simulink model "Motor_Fault_System"  (R2025b)
settings: Solver=ode4  StartTime=0.0  StopTime=30  FixedStep=0.01  RelTol=1e-3
settings Model: Creator=anifa  LastModifiedBy=anifa

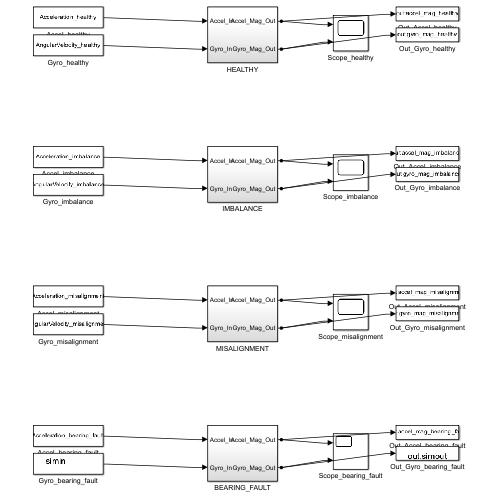
[thumbnail: Simulink's stored preview of the top-level diagram]
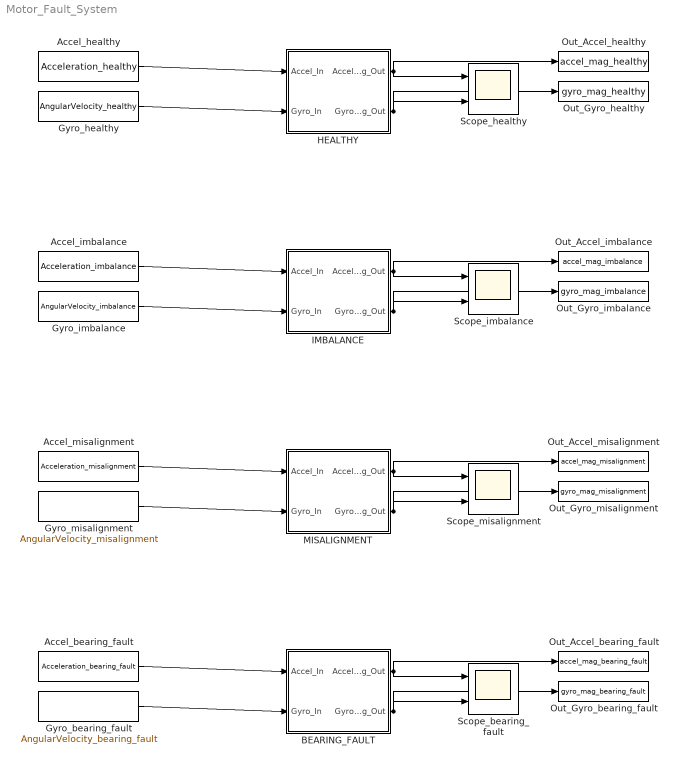
== system Motor_Fault_System ==
  Accel_bearing_fault : FromWorkspace  VariableName=Acceleration_bearing_fault
  Accel_healthy : FromWorkspace  VariableName=Acceleration_healthy
  Accel_imbalance : FromWorkspace  VariableName=Acceleration_imbalance
  Accel_misalignment : FromWorkspace  VariableName=Acceleration_misalignment
  BEARING_FAULT : Subsystem
  Gyro_bearing_fault : FromWorkspace  VariableName=AngularVelocity_bearing_fault
  Gyro_healthy : FromWorkspace  VariableName=AngularVelocity_healthy
  Gyro_imbalance : FromWorkspace  VariableName=AngularVelocity_imbalance
  Gyro_misalignment : FromWorkspace  VariableName=AngularVelocity_misalignment
  HEALTHY : Subsystem
  IMBALANCE : Subsystem
  MISALIGNMENT : Subsystem
  Out_Accel_bearing_fault : ToWorkspace  VariableName=accel_mag_bearing_fault  SampleTime=-1
  Out_Accel_healthy : ToWorkspace  VariableName=accel_mag_healthy  SampleTime=-1
  Out_Accel_imbalance : ToWorkspace  VariableName=accel_mag_imbalance  SampleTime=-1
  Out_Accel_misalignment : ToWorkspace  VariableName=accel_mag_misalignment  SampleTime=-1
  Out_Gyro_bearing_fault : ToWorkspace  VariableName=gyro_mag_bearing_fault  SampleTime=-1
  Out_Gyro_healthy : ToWorkspace  VariableName=gyro_mag_healthy  SampleTime=-1
  Out_Gyro_imbalance : ToWorkspace  VariableName=gyro_mag_imbalance  SampleTime=-1
  Out_Gyro_misalignment : ToWorkspace  VariableName=gyro_mag_misalignment  SampleTime=-1
  Scope_bearing_fault : Scope  NumInputPorts=2
  Scope_healthy : Scope  NumInputPorts=2
  Scope_imbalance : Scope  NumInputPorts=2
  Scope_misalignment : Scope  NumInputPorts=2
  wires:
  Accel_healthy/1 -> HEALTHY/1(Accel_In)
  Gyro_healthy/1 -> HEALTHY/2(Gyro_In)
  HEALTHY/1(Accel_Mag_Out) -> Scope_healthy/1, Out_Accel_healthy/1
  HEALTHY/2(Gyro_Mag_Out) -> Scope_healthy/2, Out_Gyro_healthy/1
  Accel_imbalance/1 -> IMBALANCE/1(Accel_In)
  Gyro_imbalance/1 -> IMBALANCE/2(Gyro_In)
  IMBALANCE/1(Accel_Mag_Out) -> Scope_imbalance/1, Out_Accel_imbalance/1
  IMBALANCE/2(Gyro_Mag_Out) -> Scope_imbalance/2, Out_Gyro_imbalance/1
  Accel_misalignment/1 -> MISALIGNMENT/1(Accel_In)
  Gyro_misalignment/1 -> MISALIGNMENT/2(Gyro_In)
  MISALIGNMENT/1(Accel_Mag_Out) -> Scope_misalignment/1, Out_Accel_misalignment/1
  MISALIGNMENT/2(Gyro_Mag_Out) -> Scope_misalignment/2, Out_Gyro_misalignment/1
  Accel_bearing_fault/1 -> BEARING_FAULT/1(Accel_In)
  Gyro_bearing_fault/1 -> BEARING_FAULT/2(Gyro_In)
  BEARING_FAULT/1(Accel_Mag_Out) -> Scope_bearing_fault/1, Out_Accel_bearing_fault/1
  BEARING_FAULT/2(Gyro_Mag_Out) -> Scope_bearing_fault/2, Out_Gyro_bearing_fault/1

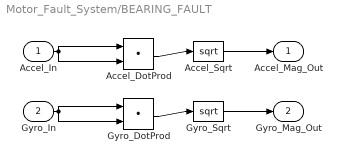
== system Motor_Fault_System/BEARING_FAULT ==
  Accel_In : Inport
  Gyro_In : Inport  Port=2
  Accel_DotProd : DotProduct  OutDataTypeStr=Inherit: Inherit via internal rule
  Accel_Sqrt : Sqrt
  Gyro_DotProd : DotProduct  OutDataTypeStr=Inherit: Inherit via internal rule
  Gyro_Sqrt : Sqrt
  Accel_Mag_Out : Outport
  Gyro_Mag_Out : Outport  Port=2
  wires:
  Accel_In/1 -> Accel_DotProd/1, Accel_DotProd/2
  Accel_DotProd/1 -> Accel_Sqrt/1
  Accel_Sqrt/1 -> Accel_Mag_Out/1
  Gyro_In/1 -> Gyro_DotProd/1, Gyro_DotProd/2
  Gyro_DotProd/1 -> Gyro_Sqrt/1
  Gyro_Sqrt/1 -> Gyro_Mag_Out/1

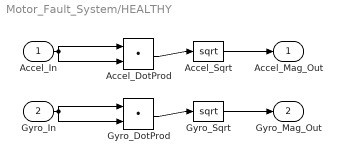
== system Motor_Fault_System/HEALTHY ==
  Accel_In : Inport
  Gyro_In : Inport  Port=2
  Accel_DotProd : DotProduct  OutDataTypeStr=Inherit: Inherit via internal rule
  Accel_Sqrt : Sqrt
  Gyro_DotProd : DotProduct  OutDataTypeStr=Inherit: Inherit via internal rule
  Gyro_Sqrt : Sqrt
  Accel_Mag_Out : Outport
  Gyro_Mag_Out : Outport  Port=2
  wires:
  Accel_In/1 -> Accel_DotProd/1, Accel_DotProd/2
  Accel_DotProd/1 -> Accel_Sqrt/1
  Accel_Sqrt/1 -> Accel_Mag_Out/1
  Gyro_In/1 -> Gyro_DotProd/1, Gyro_DotProd/2
  Gyro_DotProd/1 -> Gyro_Sqrt/1
  Gyro_Sqrt/1 -> Gyro_Mag_Out/1

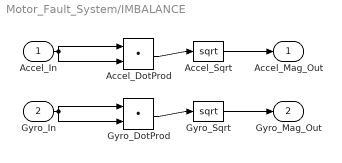
== system Motor_Fault_System/IMBALANCE ==
  Accel_In : Inport
  Gyro_In : Inport  Port=2
  Accel_DotProd : DotProduct  OutDataTypeStr=Inherit: Inherit via internal rule
  Accel_Sqrt : Sqrt
  Gyro_DotProd : DotProduct  OutDataTypeStr=Inherit: Inherit via internal rule
  Gyro_Sqrt : Sqrt
  Accel_Mag_Out : Outport
  Gyro_Mag_Out : Outport  Port=2
  wires:
  Accel_In/1 -> Accel_DotProd/1, Accel_DotProd/2
  Accel_DotProd/1 -> Accel_Sqrt/1
  Accel_Sqrt/1 -> Accel_Mag_Out/1
  Gyro_In/1 -> Gyro_DotProd/1, Gyro_DotProd/2
  Gyro_DotProd/1 -> Gyro_Sqrt/1
  Gyro_Sqrt/1 -> Gyro_Mag_Out/1

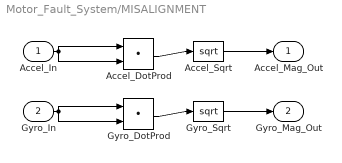
== system Motor_Fault_System/MISALIGNMENT ==
  Accel_In : Inport
  Gyro_In : Inport  Port=2
  Accel_DotProd : DotProduct  OutDataTypeStr=Inherit: Inherit via internal rule
  Accel_Sqrt : Sqrt
  Gyro_DotProd : DotProduct  OutDataTypeStr=Inherit: Inherit via internal rule
  Gyro_Sqrt : Sqrt
  Accel_Mag_Out : Outport
  Gyro_Mag_Out : Outport  Port=2
  wires:
  Accel_In/1 -> Accel_DotProd/1, Accel_DotProd/2
  Accel_DotProd/1 -> Accel_Sqrt/1
  Accel_Sqrt/1 -> Accel_Mag_Out/1
  Gyro_In/1 -> Gyro_DotProd/1, Gyro_DotProd/2
  Gyro_DotProd/1 -> Gyro_Sqrt/1
  Gyro_Sqrt/1 -> Gyro_Mag_Out/1
